simulink model "mnist_softmax_adam"  (R2017a)
settings: Solver=FixedStepDiscrete  StartTime=0.0  StopTime=1000  FixedStep=1  RelTol=1e-3
libraries: ad_blocks x10, simulink x4, dspindex x1
settings Model: PauseTimes=2  SnapshotBufferSize=2  SnapshotInterval=1  Creator=percro2  LastModifiedBy=eruffaldi

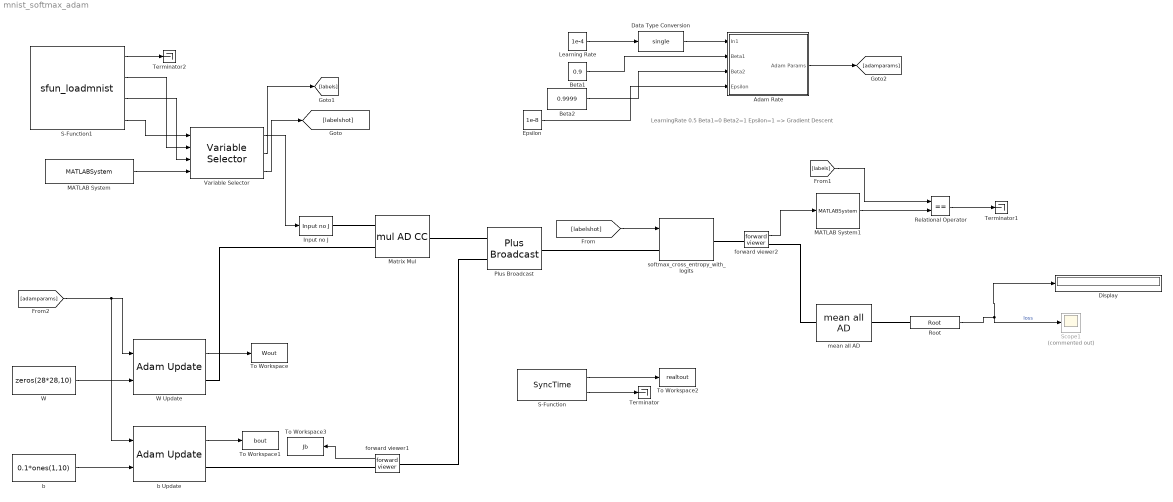
== system mnist_softmax_adam ==
  note: LearningRate 0.5 Beta1=0 Beta2=1 Epsilon=1 => Gradient Descent
  Adam Rate : Subsystem
  Beta1 : Constant  Value=0.9
  Beta2 : Constant  Value=0.9999
  Data Type Conversion : DataTypeConversion  OutDataTypeStr=single
  Display : Display
  Epsilon : Constant  Value=1e-8
  Input no J : ad_blocks/Input no J  SystemSampleTime=-1
  Learning Rate : Constant  Value=1e-4
  MATLAB System : MATLABSystem  System=MnistSystemInt  trainset=1  items=100  SimulateUsing=Interpreted execution
      mask Type: MnistSystemInt
      mask Display:
      | disp('MnistSystemInt');
      | port_label('output',1,'indices');
  MATLAB System1 : MATLABSystem  System=ArgmaxSystemD2  SimulateUsing=Code generation
      mask Type: ArgmaxSystemD2
      mask Display:
      | disp('ArgmaxSystemD2');
      | port_label('input',1,'x');
      | port_label('output',1,'y');
  Matrix Mul : ad_blocks/mul AD CC
  Plus Broadcast : ad_blocks/Plus Broadcast
  Relational Operator : RelationalOperator  Operator===  OutDataTypeStr=boolean  RndMeth=Simplest
  Root : ad_blocks/Root  Description=Top level AD block: gets the incoming value, pushes the scalar 1 gradient  SystemSampleTime=-1
  S-Function : S-Function  Priority=1024  FunctionName=SyncTime  Parameters=dt  SFunctionDeploymentMode=off  EnableBusSupport=off  mask{dt=0}
      mask prompts: dt "Period (s) or 0 for sleepless"
      mask Display:
      | port_label('output',1,'Unix Epoch s');
      | port_label('output',2,'Slept s');
  S-Function1 : S-Function  FunctionName=sfun_loadmnist  Parameters=1  SFunctionDeploymentMode=off  EnableBusSupport=off
  Scope1 : Scope  Commented=on
  Terminator : Terminator
  Terminator1 : Terminator
  Terminator2 : Terminator
  To Workspace : ToWorkspace  VariableName=Wout  SaveFormat=Timeseries  SampleTime=-1
  To Workspace1 : ToWorkspace  VariableName=bout  SaveFormat=Timeseries  SampleTime=-1
  To Workspace2 : ToWorkspace  VariableName=realtout  SaveFormat=Timeseries  SampleTime=1
  To Workspace3 : ToWorkspace  VariableName=Jb  SaveFormat=Timeseries  SampleTime=-1
  Variable Selector : dspindex/Variable Selector  NumInputs=3  rowsOrCols=Rows  IdxMode=Variable  Elements=[1 3]  ZerOneIdxMode=One-based  errmode=Generate Error  FillMode=on  FillValues=0
  W : Constant  Value=zeros(28*28,10)  OutDataTypeStr=Inherit: Inherit via back propagation
  W Update : ad_blocks/Adam Update
  b : Constant  Value=0.1*ones(1,10)  OutDataTypeStr=Inherit: Inherit via back propagation
  b Update : ad_blocks/Adam Update
  forward viewer1 : ad_blocks/forward viewer  SystemSampleTime=-1
  forward viewer2 : ad_blocks/forward viewer  SystemSampleTime=-1
  mean all AD : ad_blocks/mean all AD
  softmax_cross_entropy_with_logits : ad_blocks/softmax_cross_entropy_with_logits
  wires:
  Root/1 -> Display/1, Scope1/1  "loss"
  forward viewer2/1 -> MATLAB System1/1
  [adamparams] -> b Update/1, W Update/1
  W/1 -> W Update/2
  W Update/1 -> To Workspace/1
  b Update/1 -> To Workspace1/1
  MATLAB System1/1 -> Relational Operator/2
  [labelshot] -> softmax_cross_entropy_with_logits/1
  [labels] -> Relational Operator/1
  b/1 -> b Update/2
  Relational Operator/1 -> Terminator1/1
  S-Function/1 -> To Workspace2/1
  S-Function/2 -> Terminator/1
  Learning Rate/1 -> Data Type Conversion/1
  Adam Rate/1(Adam Params) -> [adamparams]
  forward viewer1/1 -> To Workspace3/1
  S-Function1/2 -> Variable Selector/2
  Variable Selector/2 -> [labels]
  S-Function1/3 -> Variable Selector/3
  MATLAB System/1 -> Variable Selector/4
  S-Function1/4 -> Variable Selector/1
  Variable Selector/1 -> Input no J/1
  Variable Selector/3 -> [labelshot]
  Beta1/1 -> Adam Rate/2(Beta1)
  Beta2/1 -> Adam Rate/3(Beta2)
  Epsilon/1 -> Adam Rate/4(Epsilon)
  Data Type Conversion/1 -> Adam Rate/1(In1)
  S-Function1/1 -> Terminator2/1
  connections:
  Input no J/RConn1 -- Matrix Mul/LConn1
  W Update/RConn1 -- Matrix Mul/LConn2
  Plus Broadcast/RConn1 -- softmax_cross_entropy_with_logits/LConn1
  softmax_cross_entropy_with_logits/RConn1 -- forward viewer2/LConn1
  mean all AD/RConn1 -- Root/LConn1
  forward viewer2/RConn1 -- mean all AD/LConn1
  Matrix Mul/RConn1 -- Plus Broadcast/LConn1
  Plus Broadcast/LConn2 -- forward viewer1/LConn1
  forward viewer1/RConn1 -- b Update/RConn1

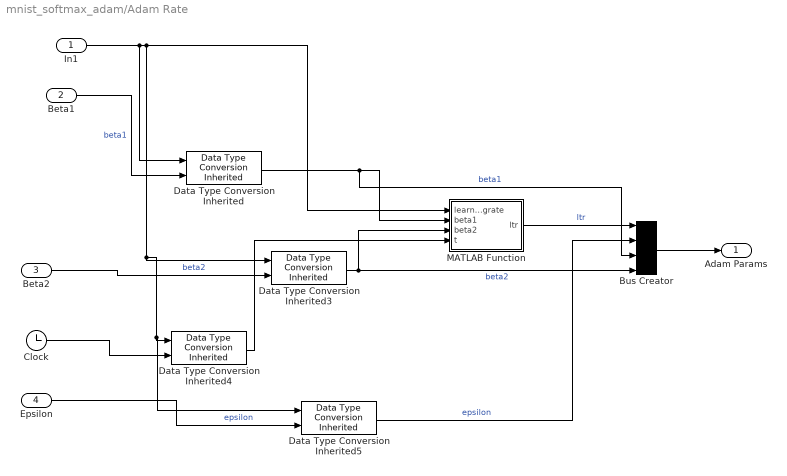
== system mnist_softmax_adam/Adam Rate ==
  In1 : Inport
  Beta1 : Inport  Port=2
  Beta2 : Inport  Port=3
  Epsilon : Inport  Port=4
  Bus Creator : BusCreator  Inputs=4
  Clock : Clock
  Data Type Conversion Inherited{,3..5} (4 alike) : simulink/Signal Attributes/Data Type Conversion Inherited  ConvertRealWorld=Real World Value  DoSatur=off
      settings: SourceProductName=Simulink  SourceProductBaseCode=SL
  MATLAB Function : MATLAB Function  TreatAsAtomicUnit=on
  Adam Params : Outport
  wires:
  MATLAB Function/1(ltr) -> Bus Creator/1  "ltr"
  Bus Creator/1 -> Adam Params/1
  Data Type Conversion Inherited/1 -> Bus Creator/3, MATLAB Function/2(beta1)  "beta1"
  In1/1 -> Data Type Conversion Inherited/1, Data Type Conversion Inherited5/1, Data Type Conversion Inherited4/1, Data Type Conversion Inherited3/1, MATLAB Function/1(learningrate)
  Beta1/1 -> Data Type Conversion Inherited/2  "beta1"
  Beta2/1 -> Data Type Conversion Inherited3/2  "beta2"
  Data Type Conversion Inherited3/1 -> MATLAB Function/3(beta2), Bus Creator/4  "beta2"
  Clock/1 -> Data Type Conversion Inherited4/2
  Data Type Conversion Inherited4/1 -> MATLAB Function/4(t)
  Epsilon/1 -> Data Type Conversion Inherited5/2  "epsilon"
  Data Type Conversion Inherited5/1 -> Bus Creator/2  "epsilon"

== matlab function mnist_softmax_adam/Adam Rate/MATLAB Function ==
  data: learningrate input; ltr output; beta1 input; beta2 input; t input
function ltr = fcn(learningrate,beta1,beta2,t)

if beta1 == 1 || beta2 == 1
    ltr = -learningrate;
else
    ltr = - learningrate * sqrt(1 - beta2^t) / (1 - beta1^t);
end
